simulink model "CiMappedEngine"  (R2018b)
settings: Solver=VariableStepAuto  StartTime=0.0  StopTime=inf  RelTol=1e-3  EnableMultiTasking=on
model workspace (MAT data in the model file):
  AccPwrbp = [0 2]
  AccSpdbp = [300 750]
  Cps = 2
  NCyl = 4
  Pstd = 101325
  Rair = 287.05
  Sinj = 6.45161290323
  TimeCnstECP = 0.125
  TimeCnstEGR = 0.125
  TimeCnstETC = 0.085
  TimeCnstICP = 0.125
  TimeCnstIVL = 0.125
  TimeCnstMFA = 0.125
  TimeCnstSWVA = 0.125
  TimeCnstVCR = 0.125
  TimeCnstVGT = 0.15
  TimeCnstVIRL = 0.125
  TimeCnstWGA = 0.15
  Tstd = 293.15
  Vd = 0.0015
  f_air = [0 0 0 0 0 0 0 0 0 0 0 0 ... (320 elements, 20x16)]
  f_co = [0 0 0 0 0 0 0 0 0 0 0 0 ... (320 elements, 20x16)]
  f_co2 = [0 0 0 0 0 0 0 0 0 0 0 0 ... (320 elements, 20x16)]
  f_eff = [0 0 0 0 0 0 0 0 0 0 0 0 ... (320 elements, 20x16)]
  f_fuel = [0 0 0 0 0 0 0 0 0 0 0 0 ... (320 elements, 20x16)]
  f_hc = [0 0 0 0 0 0 0 0 0 0 0 0 ... (320 elements, 20x16)]
  f_nox = [0 0 0 0 0 0 0 0 0 0 0 0 ... (320 elements, 20x16)]
  f_pm = [0  0  0  0  0  0  0  0  0  0  0  0  0  0  0  0; 0  0  0  0  0  0  0  0  0  0  0  0  0  0  0  0; 0  0  0  0  0  0  0  0  0  0  0  0  0  0  0  0; 0  0  0  0  0  0  0  0  0  0  0  0  0  0  0  0; 0  0  0  0  0  0  0  0  0  0  0  0  0  0  0  0; 0  0  0  0  0  0  0  0  0  0  0  0  0  0  0  0; 0  0  0  0  0  0  0  0  0  0  0  0  0  0  0  0; 0  0  0  0  0  0  0  0  0  0  0  0  0  0  0  0; 0  0  0  0  0  0  0  0  0  0  0  0  0  0  0  0; 0  0  0  0  0  0  0  0  0  0  0  0  0  0  0  0; 0  0  0  0  0  0  0  0  0  0  0  0  0  0  0  0; 0  0  0  0  0  0  0  0  0  0  0  0  0  0  0  0; 0  0  0  0  0  0  0  0  0  0  0  0  0  0  0  0; 0  0  0  0  0  0  0  0  0  0  0  0  0  0  0  0; 0  0  0  0  0  0  0  0  0  0  0  0  0  0  0  0; 0  0  0  0  0  0  0  0  0  0  0  0  0  0  0  0; 0  0  0  0  0  0  0  0  0  0  0  0  0  0  0  0; 0  0  0  0  0  0  0  0  0  0  0  0  0  0  0  0; 0  0  0  0  0  0  0  0  0  0  0  0  0  0  0  0; 0  0  0  0  0  0  0  0  0  0  0  0  0  0  0  0]
  f_tbrake = [0 1.13753137879 11.9426332722 22.7477351656 36.7347516365 52.299350938 66.4211264655 75.2678214488 82.3056067154 89.1557305474 107.57672622 127.542894583 ... (320 elements, 20x16)]
  f_tbrake_f_bpt = [0 2.63157894737 5.26315789474 7.89473684211 10.5263157895 13.1578947368 15.7894736842 18.4210526316 21.0526315789 23.6842105263 26.3157894737 28.9473684211 31.5789473684 34.2105263158 36.8421052632 39.4736842105 42.1052631579 44.7368421053 47.3684210526 50]
  f_tbrake_n_bpt = [0 1000 1285.71428571 1571.42857143 1857.14285714 2142.85714286 2428.57142857 2714.28571429 3000 3285.71428571 3571.42857143 3857.14285714 4142.85714286 4428.57142857 4714.28571429 5000]
  f_texh = [517.883201374 517.883201374 650.069530286 650.069530286 657.944120356 686.745192741 719.202605289 793.945008437 842.368962922 878.871509518 894.5166363 911.055063428 ... (320 elements, 20x16)]
libraries: autolibsharedmappedengines x1
(part 1 of 2)
settings Model: ModifiedByFormat=The MathWorks, Inc.  Creator=The MathWorks, Inc.  LastModifiedBy=The MathWorks, Inc.
settings SolverCC: DecoupledContinuousIntegration=on
settings DataIOCC: DSMLogging=off
settings DebuggingCC: LibraryContextMissingDiagnostic=none
settings SFSimCC: SimUseLocalCustomCode=off
settings RTWCC: RTWUseLocalCustomCode=off
settings CodeAppCC: StateflowObjectComments=on
settings GRTTargetCC: TargetLangStandard=C89/C90 (ANSI)
settings ConfigComp: CovMetricSettings=dsw  CovHtmlReporting=on  CovSaveCumulativeToWorkspaceVar=on  CovSaveSingleToWorkspaceVar=on  CovShowResultsExplorer=off  CovExternalEMLEnable=off
settings SimscapeCC: SimscapeNormalizeSystem=off  SimscapeNominalValues={1, 'bar'; 1, 'cm^3/s'; 1, 'bar*kg/s'; 1, 'kJ/kg'; 1, 'kW'}

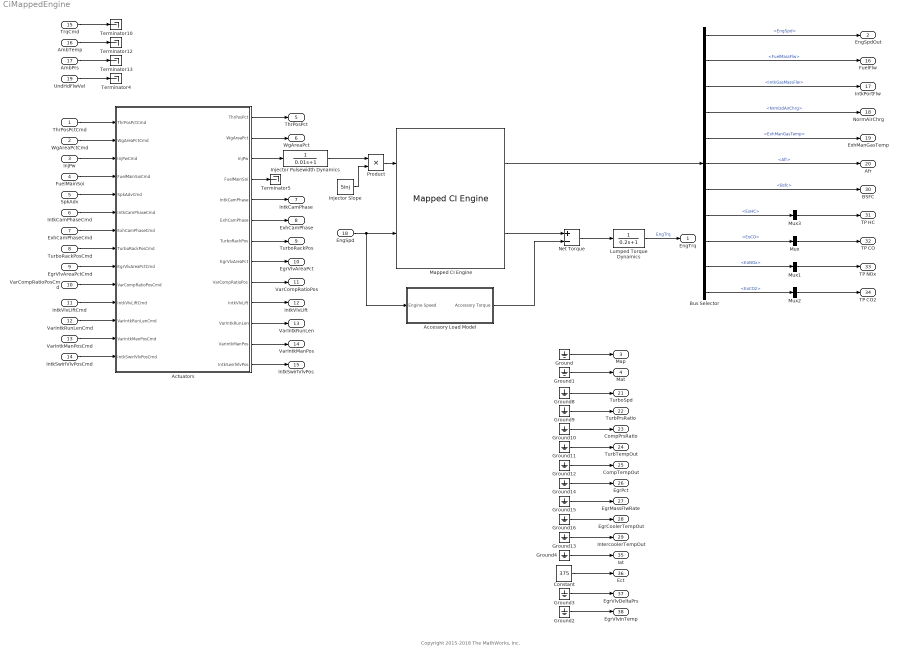
== system CiMappedEngine ==
  note: Copyright 2015-2018 The MathWorks, Inc.
  ThrPosPctCmd : Inport
  WgAreaPctCmd : Inport  Port=2
  InjPw : Inport  Port=3
  FuelMainSoi : Inport  Port=4
  SpkAdv : Inport  Port=5
  IntkCamPhaseCmd : Inport  Port=6
  ExhCamPhaseCmd : Inport  Port=7
  TurboRackPosCmd : Inport  Port=8
  EgrVlvAreaPctCmd : Inport  Port=9
  VarCompRatioPosCmd : Inport  Port=10
  IntkVlvLiftCmd : Inport  Port=11
  VarIntkRunLenCmd : Inport  Port=12
  VarIntkManPosCmd : Inport  Port=13
  IntkSwirlVlvPosCmd : Inport  Port=14
  TrqCmd : Inport  Port=15  Unit=N*m
  AmbTemp : Inport  Port=16  Unit=K
  AmbPrs : Inport  Port=17  Unit=Pa
  EngSpd : Inport  Port=18  Interpolate=off
  UndHdFlwVel : Inport  Port=19  Unit=m/s
  Accessory Load Model : Subsystem
  Actuators : Subsystem
  Bus Selector : BusSelector  OutputSignals=EngSpd,FuelMassFlw,IntkGasMassFlw,NrmlzdAirChrg,ExhManGasTemp,Afr,Bsfc,EoHC,EoCO,EoNOx,EoCO2
  Constant : Constant  Value=375
  Ground{,1..4,8..16} (14 alike) : Ground
  Injector Pulsewidth Dynamics : TransferFcn  Denominator=[0.01 1]
  Injector Slope : Constant  Value=Sinj
  Lumped Torque Dynamics : TransferFcn  Denominator=[0.2 1]
  Mapped CI Engine : autolibsharedmappedengines/Mapped CI Engine  InputCmdPopup=Fuel mass  TurboLagCheckbox=off  rowVarName=TrqCmd  f_tbrake_f_bpt=f_tbrake_f_bpt  f_tbrake_t_bpt=[0 4.017 21.26 37.37 52.22 65.88 78.77 91.44 104.2 116.8 129.3 141.4 153.4 165.7 178.4 191.7 205.6 219.7 233.5 246.7]  colVarName=EngSpd  f_tbrake_n_bpt=f_tbrake_n_bpt  NCyl=NCyl  Cps=Cps  Vd=Vd  Rair=Rair  Pstd=Pstd  Tstd=Tstd  Use1=on  Use2=on  Use3=on  Use4=on  Use5=on  Use6=on  Use7=on  Use8=on  Use9=on  Use10=off  f_tbrake_bst=[90, 95, 95, 95, 96, 100, 104, 104, 104, 100, 95, 85, 75, 67, 60, 55]  tau_nat=0.1  tau_bst_rising=1.0  tau_bst_falling=0.7  f_blend_frac=0.01  Name1=Brake Torque  f_tbrake=f_tbrake  Name2=Air Mass Flow  f_air=f_air  Name3=Fuel Flow  f_fuel=f_fuel  Name4=Exhaust Temperature  f_texh=f_texh  Name5=[300 300 300 300 300 300 300 300 300 300 300 300 300 300 300 300 300 300 300 300;297.183191911082 296.381813482439 298.389346568793 300 300 300 300 300 300 300 300 300 294.67266237158 289.737568904754 289.12856875624 291.461389167304 295.189395927038 297.348559050166 294.666946050542 286.881979097439;300 300 300 300 300 300 300 300 300 300 300 295.311694583484 288.854995920935 285.748220888279 286.130153267134 289.042144321121 293.243311010686 295.055826333218 287.545970834715 273.554783231216;300 300 300 300 298.49404534039 284.553749077953 261.448898184998 238.707345487409 254.949441131286 265.599575550091 295.677653030517 300 300 300 300 300 300 300 284.419815180476 261.388018187759;299.898205056662 292.176013706802 280.489559192747 273.801475207664 285.267789972213 268.982289185 248.031226594938 237.002933175585 247.269718357657 266.486860456224 296.010628081896 300 300 300 300 300 300 300 286.278851967763 251.317497463977;257.787117715529 230.011418991628 194.79567839807 217.609945177071 238.011497997128 244.713362579463 248.307562590703 254.695511354579 262.767152384925 269.435894142237 279.964353630393 300 300 300 300 300 300 300 300 252.247426167928;244.322164627464 226.527131172705 213.047581606847 208.860573467528 215.436572460517 230.257055418638 247.71372128472 261.030678888545 264.562685576978 255.804646726121 236.560489592442 212.844962970881 193.289036483877 186.243942541361 196.420463604227 222.426431060715 256.501420981836 286.894148423494 300 294.746256064465;219.827091553639 224.00842185519 226.545147573507 228.801538184105 231.197671510704 233.328041106659 234.425064195191 233.869076886551 231.523160498036 227.853678111254 223.908810740718 221.191949545254 221.375059646733 225.801644328901 234.876097447666 247.606442228722 261.586362170144 273.512050995951 280.050090404176 278.699668055487;253.235653200863 238.315624663681 223.001448394165 210.254255439123 202.14302656868 199.596251942444 202.290727140351 208.74083615883 216.703414841512 223.908681461858 228.900345602987 231.595168993526 233.230095692023 235.664906994489 240.366291593439 247.574154702973 256.032407983205 263.350862590025 266.765300968141 263.943316381967;248.250293366452 233.417397015265 222.629357327487 216.596802702064 214.504013108419 214.81806354172 216.051223315593 217.193946153414 217.807532354882 217.934808981726 217.977570533706 218.581966234929 220.499755224279 224.409471192001 230.735069374117 239.511489718516 250.303231623288 262.14379859624 273.489242792845 282.252586128849;242.086120224848 231.058285918819 223.245524598864 216.337716642453 212.00473270881 210.686778459967 211.585047714386 213.166686160244 214.004603934158 213.551990844805 212.439775437554 212.136104170727 214.180677075341 219.45152567214 227.861873339277 238.565025705036 250.403923777452 262.226566009688 272.865736774747 280.895220351927;240.36005533725 232.486162829539 226.900934366509 218.228275058477 210.073138425769 205.914056262523 206.863704975026 211.780406579307 218.363100263461 224.502124938947 229.114817814123 232.147403860389 234.026061788487 235.150186450836 235.841184590216 236.675239999685 238.744779946964 243.413612851756 251.528383016844 262.510332308677;239.698447912074 232.198026859744 223.919414459446 215.521411204134 208.833017267823 206.211824916001 207.251476971107 209.476538949511 210.219164042317 208.589475472156 206.308833127149 206.824526287407 213.201356834861 226.090216081071 243.04996560855 259.64415199246 271.618523010977 276.830575274702 275.838901872999 270.954993619848;239.699124464556 233.605232579107 228.311199393793 224.353241232463 217.305414394382 214.392354260996 217.338892875621 224.705113920913 232.919686598668 238.298745155624 238.931493145234 235.439120293715 230.335964150791 226.556951715392 226.115112416361 229.595190701737 236.519242380678 246.043219412989 257.344197449557 263.377380468519;239.816295103623 235.306294052789 231.603067258988 227.141295414711 219.929221129055 221.663517863192 223.173313363379 ...(+1903 chars)]  f_eff=f_eff  Name6=EO HC  f_hc=f_hc  Name7=EO CO  f_co=f_co  Name8=EO NOx  f_nox=f_nox  Name9=EO CO2  f_co2=f_co2  Name10=Brake Torque  f_pm=f_pm  aMode=1  CalMapsFuelCmdData={'', '', 'MappedEngine-Torque', 'MappedEngine-Nonfiring'}  CalMapsTrqCmdData={'', '', 'MappedEngine-Torque', 'MappedEngine-Nonfiring'}
      settings: SourceProductName=Powertrain Blockset  SourceProductBaseCode=PW
  Mux{,1..3} (4 alike) : Mux  Inputs=1
  Net Torque : Sum  Inputs=+-
  Product : Product
  Terminator{4..5,10,12..13} (5 alike) : Terminator
  EngTrq : Outport  Unit=N*m
  EngSpdOut : Outport  Port=2
  Map : Outport  Port=3  Unit=Pa
  Mat : Outport  Port=4  Unit=K
  ThrPosPct : Outport  Port=5
  WgAreaPct : Outport  Port=6
  IntkCamPhase : Outport  Port=7
  ExhCamPhase : Outport  Port=8
  TurboRackPos : Outport  Port=9
  EgrVlvAreaPct : Outport  Port=10
  VarCompRatioPos : Outport  Port=11
  IntkVlvLift : Outport  Port=12
  VarIntkRunLen : Outport  Port=13
  VarIntkManPos : Outport  Port=14
  IntkSwirlVlvPos : Outport  Port=15
  FuelFlw : Outport  Port=16
  IntkPortFlw : Outport  Port=17
  NormAirChrg : Outport  Port=18
  ExhManGasTemp : Outport  Port=19
  Afr : Outport  Port=20
  TurboSpd : Outport  Port=21  Unit=rad/s
  TurbPrsRatio : Outport  Port=22  Unit=1
  CompPrsRatio : Outport  Port=23  Unit=1
  TurbTempOut : Outport  Port=24  Unit=K
  CompTempOut : Outport  Port=25  Unit=K
  EgrPct : Outport  Port=26  Unit=%
  EgrMassFlwRate : Outport  Port=27  Unit=kg/s
  EgrCoolerTempOut : Outport  Port=28  Unit=K
  IntercoolerTempOut : Outport  Port=29  Unit=K
  BSFC : Outport  Port=30
  TP HC : Outport  Port=31
  TP CO : Outport  Port=32
  TP NOx : Outport  Port=33
  TP CO2 : Outport  Port=34
  Iat : Outport  Port=35  Unit=K
  Ect : Outport  Port=36  Unit=K
  EgrVlvDeltaPrs : Outport  Port=37  Unit=Pa
  EgrVlvInTemp : Outport  Port=38  Unit=K
  wires:
  InjPw/1 -> Actuators/3(InjPwCmd)
  EngSpd/1 -> Accessory Load Model/1(Engine Speed), Mapped CI Engine/2
  Mapped CI Engine/2 -> Net Torque/1
  Accessory Load Model/1(Accessory Torque) -> Net Torque/2
  Lumped Torque Dynamics/1 -> EngTrq/1  "EngTrq"
  Product/1 -> Mapped CI Engine/1
  Injector Slope/1 -> Product/2
  Net Torque/1 -> Lumped Torque Dynamics/1
  AmbTemp/1 -> Terminator12/1
  Mapped CI Engine/1 -> Bus Selector/1
  Ground/1 -> Map/1
  Ground1/1 -> Mat/1
  TrqCmd/1 -> Terminator10/1
  AmbPrs/1 -> Terminator13/1
  UndHdFlwVel/1 -> Terminator4/1
  Bus Selector/5 -> ExhManGasTemp/1  "<ExhManGasTemp>"
  Bus Selector/6 -> Afr/1  "<Afr>"
  Bus Selector/1 -> EngSpdOut/1  "<EngSpd>"
  Bus Selector/2 -> FuelFlw/1  "<FuelMassFlw>"
  Bus Selector/3 -> IntkPortFlw/1  "<IntkGasMassFlw>"
  Bus Selector/8 -> Mux3/1  "<EoHC>"
  Bus Selector/9 -> Mux/1  "<EoCO>"
  Bus Selector/10 -> Mux1/1  "<EoNOx>"
  Bus Selector/11 -> Mux2/1  "<EoCO2>"
  Mux3/1 -> TP HC/1
  Mux/1 -> TP CO/1
  Mux1/1 -> TP NOx/1
  Mux2/1 -> TP CO2/1
  Bus Selector/7 -> BSFC/1  "<Bsfc>"
  Bus Selector/4 -> NormAirChrg/1  "<NrmlzdAirChrg>"
  Ground8/1 -> TurboSpd/1
  Ground9/1 -> TurbPrsRatio/1
  Ground10/1 -> CompPrsRatio/1
  Ground11/1 -> TurbTempOut/1
  Ground12/1 -> CompTempOut/1
  Ground13/1 -> IntercoolerTempOut/1
  Ground14/1 -> EgrPct/1
  Ground15/1 -> EgrMassFlwRate/1
  Ground16/1 -> EgrCoolerTempOut/1
  Injector Pulsewidth Dynamics/1 -> Product/1
  ThrPosPctCmd/1 -> Actuators/1(ThrPosPctCmd)
  WgAreaPctCmd/1 -> Actuators/2(WgAreaPctCmd)
  Actuators/3(InjPw) -> Injector Pulsewidth Dynamics/1
  Actuators/1(ThrPosPct) -> ThrPosPct/1
  Actuators/2(WgAreaPct) -> WgAreaPct/1
  Actuators/4(FuelMainSoi) -> Terminator5/1
  FuelMainSoi/1 -> Actuators/4(FuelMainSoiCmd)
  SpkAdv/1 -> Actuators/5(SpkAdvCmd)
  IntkCamPhaseCmd/1 -> Actuators/6(IntkCamPhaseCmd)
  ExhCamPhaseCmd/1 -> Actuators/7(ExhCamPhaseCmd)
  TurboRackPosCmd/1 -> Actuators/8(TurboRackPosCmd)
  EgrVlvAreaPctCmd/1 -> Actuators/9(EgrVlvAreaPctCmd)
  VarCompRatioPosCmd/1 -> Actuators/10(VarCompRatioPosCmd)
  IntkVlvLiftCmd/1 -> Actuators/11(IntkVlvLiftCmd)
  VarIntkRunLenCmd/1 -> Actuators/12(VarIntkRunLenCmd)
  VarIntkManPosCmd/1 -> Actuators/13(VarIntkManPosCmd)
  IntkSwirlVlvPosCmd/1 -> Actuators/14(IntkSwirlVlvPosCmd)
  Actuators/13(IntkSwirlVlvPos) -> IntkSwirlVlvPos/1
  Actuators/12(VarIntkManPos) -> VarIntkManPos/1
  Actuators/10(IntkVlvLift) -> IntkVlvLift/1
  Actuators/9(VarCompRatioPos) -> VarCompRatioPos/1
  Actuators/8(EgrVlvAreaPct) -> EgrVlvAreaPct/1
  Actuators/7(TurboRackPos) -> TurboRackPos/1
  Actuators/6(ExhCamPhase) -> ExhCamPhase/1
  Actuators/5(IntkCamPhase) -> IntkCamPhase/1
  Actuators/11(VarIntkRunLen) -> VarIntkRunLen/1
  Constant/1 -> Ect/1
  Ground3/1 -> EgrVlvDeltaPrs/1
  Ground2/1 -> EgrVlvInTemp/1
  Ground4/1 -> Iat/1
